simulink model "week1problem8"  (R2020b)
settings: Solver=VariableStepAuto  StartTime=0.0  StopTime=10.0  RelTol=1e-3
settings Model: Creator=admin  LastModifiedBy=admin

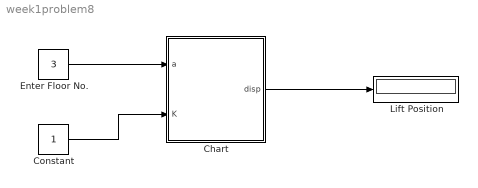
== system week1problem8 ==
  Chart : Stateflow chart  TreatAsAtomicUnit=on
  Constant : Constant
  Enter Floor No. : Constant  Value=3
  Lift Position : Display
  wires:
  Chart/1(disp) -> Lift Position/1
  Enter Floor No./1 -> Chart/1(a)
  Constant/1 -> Chart/2(K)

== stateflow chart week1problem8/Chart ==
  state ElevatorMode [parallel]
    settings: executionOrder=1
    state FifthF
      en:
      disp=5;
    state FourthF
      en:
      disp=4;
    state ThirdF
      en:
      disp=3;
    state SecondF
      en:
      disp=2;
    state FirstF
      en:
      disp=1;
    state GroundF
      en:
      disp=0;
    FourthF -> FifthF [order 2] : [a>4 && K==1]
    FifthF -> FourthF : [eve==1]
    ThirdF -> FourthF [order 1] : [a>3 && K==1]
    FourthF -> ThirdF [order 1] : [eve==1]
    SecondF -> ThirdF [order 1] : [a>2 && K==1]
    ThirdF -> SecondF [order 2] : [eve==1]
    FirstF -> SecondF [order 1] : [a>1 && K==1]
    SecondF -> FirstF [order 2] : [eve==1]
    GroundF -> FirstF : [a >0 && K==1]
    FirstF -> GroundF [order 2] : [eve==1]
    (default) -> GroundF
  state PowerMode [parallel]
    settings: executionOrder=2
    state ActiveState
      entry:
      power=1;
      exit:
    state IdleState
      entry:
      power=0;
      exit:
    (default) -> ActiveState : {power=1}
    ActiveState -> IdleState
    IdleState -> ActiveState
  data: a input; disp output; power local; K input
  events: eve local FUNCTION_CALL_EVENT
